simulink model "HILClimbers_Integrated_V7"  (R2021a)
settings: Solver=FixedStepAuto  StartTime=0.0  StopTime=10.0  RelTol=1e-3
undefined symbols (not defined in the file or in its folder): sigbuilder_block
settings Model: VariantConfigurationObject=test_mode  TunableVars=time_period  TunableVarsStorageClass=ExportedGlobal  OrderedModelArguments=off  Creator=achu  LastModifiedBy=achu
settings DebuggingCC: AlgebraicLoopMsg=none

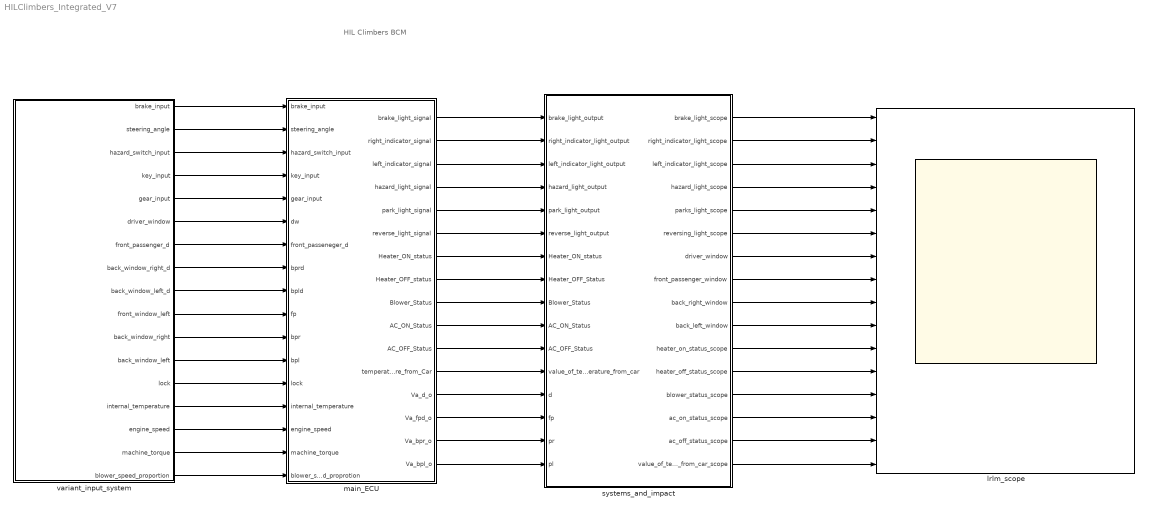
== system HILClimbers_Integrated_V7 ==
  note: HIL Climbers BCM
  lrlm_scope : Scope  NumInputPorts=16
  main_ECU : Subsystem
  systems_and_impact : Subsystem
  variant_input_system : Subsystem  InitFcn=|  Variant=on
      | manual_test=Simulink.Variant("test_mode==0");
      | automated_test=Simulink.Variant("test_mode==1");
  wires:
  systems_and_impact/4(hazard_light_scope) -> lrlm_scope/4
  systems_and_impact/12(heater_off_status_scope) -> lrlm_scope/12
  main_ECU/13(Va_d_o) -> systems_and_impact/13(d)
  systems_and_impact/10(back_left_window) -> lrlm_scope/10
  variant_input_system/6(driver_window) -> main_ECU/6(dw)
  variant_input_system/11(back_window_right) -> main_ECU/11(bpr)
  variant_input_system/9(back_window_left_d) -> main_ECU/9(bpld)
  variant_input_system/1(brake_input) -> main_ECU/1(brake_input)
  variant_input_system/10(front_window_left) -> main_ECU/10(fp)
  variant_input_system/16(machine_torque) -> main_ECU/16(machine_torque)
  variant_input_system/3(hazard_switch_input) -> main_ECU/3(hazard_switch_input)
  main_ECU/8(Heater_OFF_status) -> systems_and_impact/8(Heater_OFF_Status)
  variant_input_system/8(back_window_right_d) -> main_ECU/8(bprd)
  systems_and_impact/13(blower_status_scope) -> lrlm_scope/13
  systems_and_impact/6(reversing_light_scope) -> lrlm_scope/6
  main_ECU/3(left_indicator_signal) -> systems_and_impact/3(left_indicator_light_output)
  main_ECU/2(right_indicator_signal) -> systems_and_impact/2(right_indicator_light_output)
  variant_input_system/17(blower_speed_proportion) -> main_ECU/17(blower_speed_proprotion)
  main_ECU/10(AC_ON_Status) -> systems_and_impact/10(AC_ON_Status)
  variant_input_system/15(engine_speed) -> main_ECU/15(engine_speed)
  main_ECU/12(temperature_from_Car) -> systems_and_impact/12(value_of_temperature_from_car)
  systems_and_impact/11(heater_on_status_scope) -> lrlm_scope/11
  variant_input_system/7(front_passenger_d) -> main_ECU/7(front_passeneger_d)
  variant_input_system/13(lock) -> main_ECU/13(lock)
  systems_and_impact/16(value_of_temperature_from_car_scope) -> lrlm_scope/16
  main_ECU/9(Blower_Status) -> systems_and_impact/9(Blower_Status)
  systems_and_impact/15(ac_off_status_scope) -> lrlm_scope/15
  systems_and_impact/3(left_indicator_light_scope) -> lrlm_scope/3
  main_ECU/4(hazard_light_signal) -> systems_and_impact/4(hazard_light_output)
  main_ECU/16(Va_bpl_o) -> systems_and_impact/16(pl)
  main_ECU/11(AC_OFF_Status) -> systems_and_impact/11(AC_OFF_Status)
  main_ECU/6(reverse_light_signal) -> systems_and_impact/6(reverse_light_output)
  main_ECU/15(Va_bpr_o) -> systems_and_impact/15(pr)
  systems_and_impact/9(back_right_window) -> lrlm_scope/9
  main_ECU/7(Heater_ON_status) -> systems_and_impact/7(Heater_ON_status)
  systems_and_impact/2(right_indicator_light_scope) -> lrlm_scope/2
  variant_input_system/12(back_window_left) -> main_ECU/12(bpl)
  variant_input_system/4(key_input) -> main_ECU/4(key_input)
  systems_and_impact/8(front_passenger_window) -> lrlm_scope/8
  systems_and_impact/1(brake_light_scope) -> lrlm_scope/1
  systems_and_impact/7(driver_window) -> lrlm_scope/7
  main_ECU/1(brake_light_signal) -> systems_and_impact/1(brake_light_output)
  systems_and_impact/5(parks_light_scope) -> lrlm_scope/5
  variant_input_system/2(steering_angle) -> main_ECU/2(steering_angle)
  systems_and_impact/14(ac_on_status_scope) -> lrlm_scope/14
  main_ECU/14(Va_fpd_o) -> systems_and_impact/14(fp)
  variant_input_system/5(gear_input) -> main_ECU/5(gear_input)
  variant_input_system/14(internal_temperature) -> main_ECU/14(internal_temperature)
  main_ECU/5(park_light_signal) -> systems_and_impact/5(park_light_output)

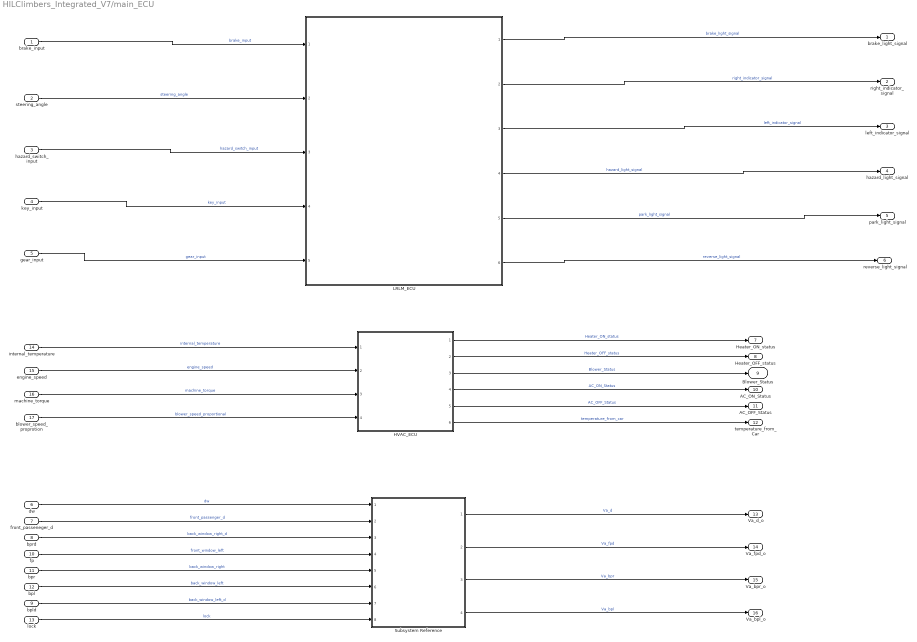
== system HILClimbers_Integrated_V7/main_ECU ==
  brake_input : Inport
  steering_angle : Inport  Port=2
  hazard_switch_input : Inport  Port=3
  key_input : Inport  Port=4
  gear_input : Inport  Port=5
  dw : Inport  Port=6
  front_passeneger_d : Inport  Port=7
  bprd : Inport  Port=8
  bpld : Inport  Port=9
  fp : Inport  Port=10
  bpr : Inport  Port=11
  bpl : Inport  Port=12
  lock : Inport  Port=13
  internal_temperature : Inport  Port=14
  engine_speed : Inport  Port=15
  machine_torque : Inport  Port=16
  blower_speed_proprotion : Inport  Port=17
  HVAC_ECU : Subsystem  ReferencedSubsystem=V6_ECU
  LRLM_ECU : Subsystem  ReferencedSubsystem=LRLM_ECU
  Subsystem Reference : Subsystem  ReferencedSubsystem=power_windows_ECU_V6
  brake_light_signal : Outport
  right_indicator_signal : Outport  Port=2
  left_indicator_signal : Outport  Port=3
  hazard_light_signal : Outport  Port=4
  park_light_signal : Outport  Port=5
  reverse_light_signal : Outport  Port=6
  Heater_ON_status : Outport  Port=7
  Heater_OFF_status : Outport  Port=8
  Blower_Status : Outport  Port=9
  AC_ON_Status : Outport  Port=10
  AC_OFF_Status : Outport  Port=11
  temperature_from_Car : Outport  Port=12
  Va_d_o : Outport  Port=13
  Va_fpd_o : Outport  Port=14
  Va_bpr_o : Outport  Port=15
  Va_bpl_o : Outport  Port=16
  wires:
  HVAC_ECU/1 -> Heater_ON_status/1  "Heater_ON_status"
  hazard_switch_input/1 -> LRLM_ECU/3  "hazard_switch_input"
  LRLM_ECU/1 -> brake_light_signal/1  "brake_light_signal"
  HVAC_ECU/5 -> AC_OFF_Status/1  "AC_OFF_Status"
  steering_angle/1 -> LRLM_ECU/2  "steering_angle"
  LRLM_ECU/2 -> right_indicator_signal/1  "right_indicator_signal"
  LRLM_ECU/5 -> park_light_signal/1  "park_light_signal"
  brake_input/1 -> LRLM_ECU/1  "brake_input"
  engine_speed/1 -> HVAC_ECU/2  "engine_speed"
  LRLM_ECU/3 -> left_indicator_signal/1  "left_indicator_signal"
  LRLM_ECU/4 -> hazard_light_signal/1  "hazard_light_signal"
  internal_temperature/1 -> HVAC_ECU/1  "internal_temperature"
  LRLM_ECU/6 -> reverse_light_signal/1  "reverse_light_signal"
  gear_input/1 -> LRLM_ECU/5  "gear_input"
  HVAC_ECU/2 -> Heater_OFF_status/1  "Heater_OFF_status"
  key_input/1 -> LRLM_ECU/4  "key_input"
  blower_speed_proprotion/1 -> HVAC_ECU/4  "blower_speed_proportional"
  HVAC_ECU/6 -> temperature_from_Car/1  "temperature_from_car"
  HVAC_ECU/4 -> AC_ON_Status/1  "AC_ON_Status"
  machine_torque/1 -> HVAC_ECU/3  "machine_torque"
  HVAC_ECU/3 -> Blower_Status/1  "Blower_Status"
  Subsystem Reference/1 -> Va_d_o/1  "Va_d"
  bpl/1 -> Subsystem Reference/6  "back_window_left"
  Subsystem Reference/3 -> Va_bpr_o/1  "Va_bpr"
  bpld/1 -> Subsystem Reference/7  "back_window_left_d"
  bprd/1 -> Subsystem Reference/3  "back_window_right_d"
  fp/1 -> Subsystem Reference/4  "front_window_left"
  Subsystem Reference/2 -> Va_fpd_o/1  "Va_fpd"
  bpr/1 -> Subsystem Reference/5  "back_window_right"
  dw/1 -> Subsystem Reference/1  "dw"
  Subsystem Reference/4 -> Va_bpl_o/1  "Va_bpl"
  lock/1 -> Subsystem Reference/8  "lock"
  front_passeneger_d/1 -> Subsystem Reference/2  "front_passenger_d"

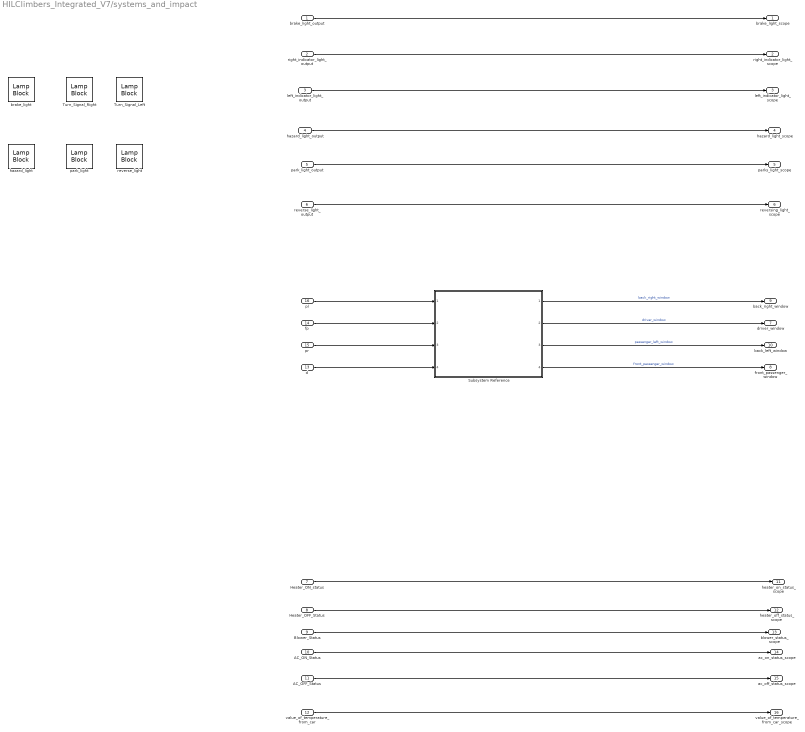
== system HILClimbers_Integrated_V7/systems_and_impact ==
  brake_light_output : Inport
  right_indicator_light_output : Inport  Port=2
  left_indicator_light_output : Inport  Port=3
  hazard_light_output : Inport  Port=4
  park_light_output : Inport  Port=5
  reverse_light_output : Inport  Port=6
  Heater_ON_status : Inport  Port=7
  Heater_OFF_Status : Inport  Port=8
  Blower_Status : Inport  Port=9
  AC_ON_Status : Inport  Port=10
  AC_OFF_Status : Inport  Port=11
  value_of_temperature_from_car : Inport  Port=12
  d : Inport  Port=13
  fp : Inport  Port=14
  pr : Inport  Port=15
  pl : Inport  Port=16
  Subsystem Reference : Subsystem  ReferencedSubsystem=power_window_system_impact_V6
  Turn_Signal_Left : LampBlock  LabelPosition=Hide  Icon=TurnSignalLeft
  Turn_Signal_Right : LampBlock  LabelPosition=Hide  Icon=TurnSignalRight
  brake_light : LampBlock  LabelPosition=Hide  Icon=LightingSwitch
  hazard_light : LampBlock  LabelPosition=Hide  Icon=Hazards
  park_light : LampBlock  LabelPosition=Hide  Icon=ParkingAssistance
  reverse_light : LampBlock  LabelPosition=Hide  Icon=RearFogLight
  brake_light_scope : Outport
  right_indicator_light_scope : Outport  Port=2
  left_indicator_light_scope : Outport  Port=3
  hazard_light_scope : Outport  Port=4
  parks_light_scope : Outport  Port=5
  reversing_light_scope : Outport  Port=6
  driver_window : Outport  Port=7
  front_passenger_window : Outport  Port=8
  back_right_window : Outport  Port=9
  back_left_window : Outport  Port=10
  heater_on_status_scope : Outport  Port=11
  heater_off_status_scope : Outport  Port=12
  blower_status_scope : Outport  Port=13
  ac_on_status_scope : Outport  Port=14
  ac_off_status_scope : Outport  Port=15
  value_of_temperature_from_car_scope : Outport  Port=16
  wires:
  hazard_light_output/1 -> hazard_light_scope/1
  reverse_light_output/1 -> reversing_light_scope/1
  park_light_output/1 -> parks_light_scope/1
  left_indicator_light_output/1 -> left_indicator_light_scope/1
  right_indicator_light_output/1 -> right_indicator_light_scope/1
  brake_light_output/1 -> brake_light_scope/1
  Subsystem Reference/4 -> front_passenger_window/1  "front_passenger_window"
  Subsystem Reference/3 -> back_left_window/1  "passenger_left_window"
  Subsystem Reference/1 -> back_right_window/1  "back_right_window"
  Subsystem Reference/2 -> driver_window/1  "driver_window"
  Blower_Status/1 -> blower_status_scope/1
  AC_OFF_Status/1 -> ac_off_status_scope/1
  AC_ON_Status/1 -> ac_on_status_scope/1
  Heater_OFF_Status/1 -> heater_off_status_scope/1
  Heater_ON_status/1 -> heater_on_status_scope/1
  value_of_temperature_from_car/1 -> value_of_temperature_from_car_scope/1
  pl/1 -> Subsystem Reference/1
  fp/1 -> Subsystem Reference/2
  d/1 -> Subsystem Reference/4
  pr/1 -> Subsystem Reference/3

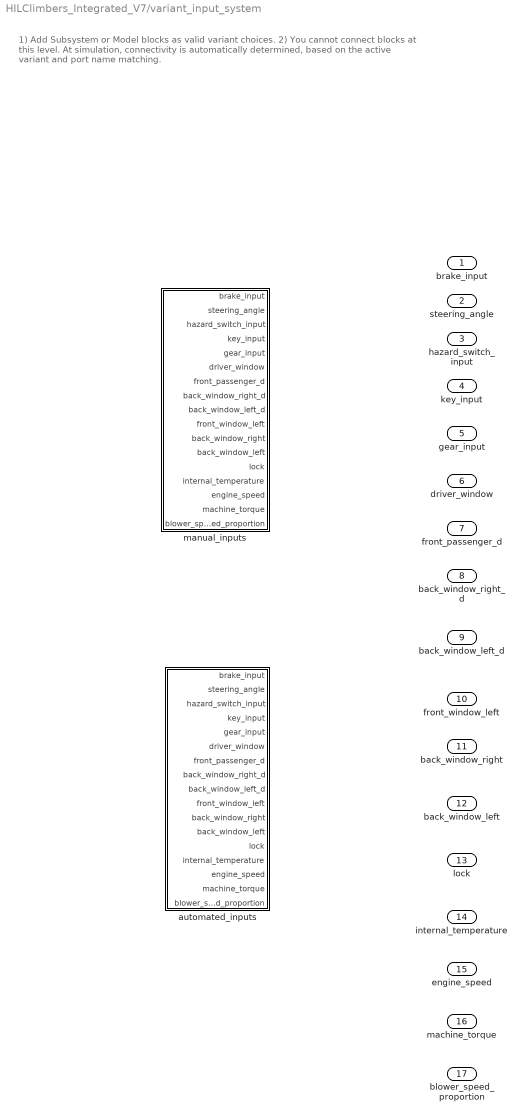
== system HILClimbers_Integrated_V7/variant_input_system ==
  note: 1) Add Subsystem or Model blocks as valid variant choices.
      | 2) You cannot connect blocks at this level. At simulation, connectivity is automatically
      | determined, based on the active variant and port name matching.
  automated_inputs : Subsystem  VariantControl=automated_test
  manual_inputs : Subsystem  VariantControl=manual_test
  brake_input : Outport
  steering_angle : Outport  Port=2
  hazard_switch_input : Outport  Port=3
  key_input : Outport  Port=4
  gear_input : Outport  Port=5
  driver_window : Outport  Port=6
  front_passenger_d : Outport  Port=7
  back_window_right_d : Outport  Port=8
  back_window_left_d : Outport  Port=9
  front_window_left : Outport  Port=10
  back_window_right : Outport  Port=11
  back_window_left : Outport  Port=12
  lock : Outport  Port=13
  internal_temperature : Outport  Port=14
  engine_speed : Outport  Port=15
  machine_torque : Outport  Port=16
  blower_speed_proportion : Outport  Port=17

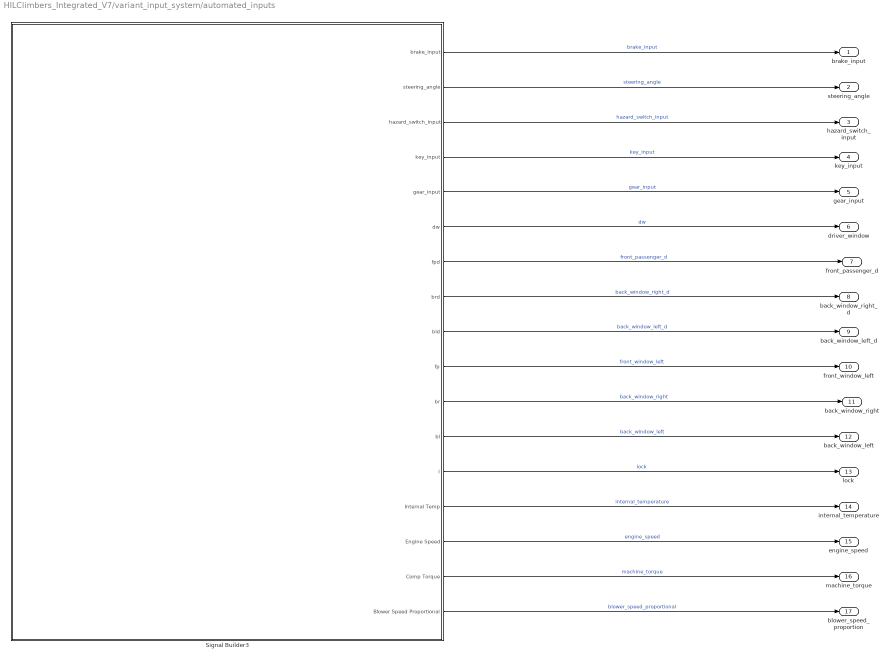
== system HILClimbers_Integrated_V7/variant_input_system/automated_inputs ==
  Signal Builder3 : Subsystem  Tag=STV Subsys  LoadFcn=sigbuilder_block('load');  StartFcn=sigbuilder_block('start');  StopFcn=sigbuilder_block('stop');  ClipboardFcn=sigbuilder_block('clipboard');  mask(Sigbuilder block){tuvar=[0:10]}
      mask help: Simulink:masks:SigbuilderBlock_MD
      mask init:
      | if ~strcmp(get_param(bdroot(gcbh),'SimulationStatus'),'stopped') tuvar = sigbuilder_block('maskInit'); end
      settings: CopyFcn=sigbuilder_block('copy');  DeleteFcn=sigbuilder_block('delete');  ModelCloseFcn=sigbuilder_block('modelClose');  PreSaveFcn=sigbuilder_block('preSave');  PauseFcn=sigbuilder_block('pause');  ContinueFcn=sigbuilder_block('continue');  NameChangeFcn=sigbuilder_block('namechange');  OpenFcn=sigbuilder_block('open',[437.6 199.2 550.4 400 ]);  CloseFcn=sigbuilder_block('close');
      mask Display: plot(0, 0, 100, 100,[2, 2, 32, 32, 2], [68, 8, 8, 68, 68],[32, 2], [38, 38], [32, 19, 2],[53, 60, 44], [32, 17, 17, 2],[16, 16, 31, 31]);txt = getActiveGroup(gcbh);text(2, 100, txt,'verticalAlignment', 'top');
  brake_input : Outport
  steering_angle : Outport  Port=2
  hazard_switch_input : Outport  Port=3
  key_input : Outport  Port=4
  gear_input : Outport  Port=5
  driver_window : Outport  Port=6
  front_passenger_d : Outport  Port=7
  back_window_right_d : Outport  Port=8
  back_window_left_d : Outport  Port=9
  front_window_left : Outport  Port=10
  back_window_right : Outport  Port=11
  back_window_left : Outport  Port=12
  lock : Outport  Port=13
  internal_temperature : Outport  Port=14
  engine_speed : Outport  Port=15
  machine_torque : Outport  Port=16
  blower_speed_proportion : Outport  Port=17
  wires:
  Signal Builder3/11(br) -> back_window_right/1  "back_window_right"
  Signal Builder3/2(steering_angle) -> steering_angle/1  "steering_angle"
  Signal Builder3/13(l) -> lock/1  "lock"
  Signal Builder3/16(Comp Torque) -> machine_torque/1  "machine_torque"
  Signal Builder3/10(fp) -> front_window_left/1  "front_window_left"
  Signal Builder3/5(gear_input) -> gear_input/1  "gear_input"
  Signal Builder3/12(bl) -> back_window_left/1  "back_window_left"
  Signal Builder3/17(Blower Speed Proportional) -> blower_speed_proportion/1  "blower_speed_proportional"
  Signal Builder3/8(brd) -> back_window_right_d/1  "back_window_right_d"
  Signal Builder3/14(Internal Temp) -> internal_temperature/1  "internal_temperature"
  Signal Builder3/3(hazard_switch_input) -> hazard_switch_input/1  "hazard_switch_input"
  Signal Builder3/6(dw) -> driver_window/1  "dw"
  Signal Builder3/1(brake_input) -> brake_input/1  "brake_input"
  Signal Builder3/7(fpd) -> front_passenger_d/1  "front_passenger_d"
  Signal Builder3/9(bld) -> back_window_left_d/1  "back_window_left_d"
  Signal Builder3/15(Engine Speed) -> engine_speed/1  "engine_speed"
  Signal Builder3/4(key_input) -> key_input/1  "key_input"

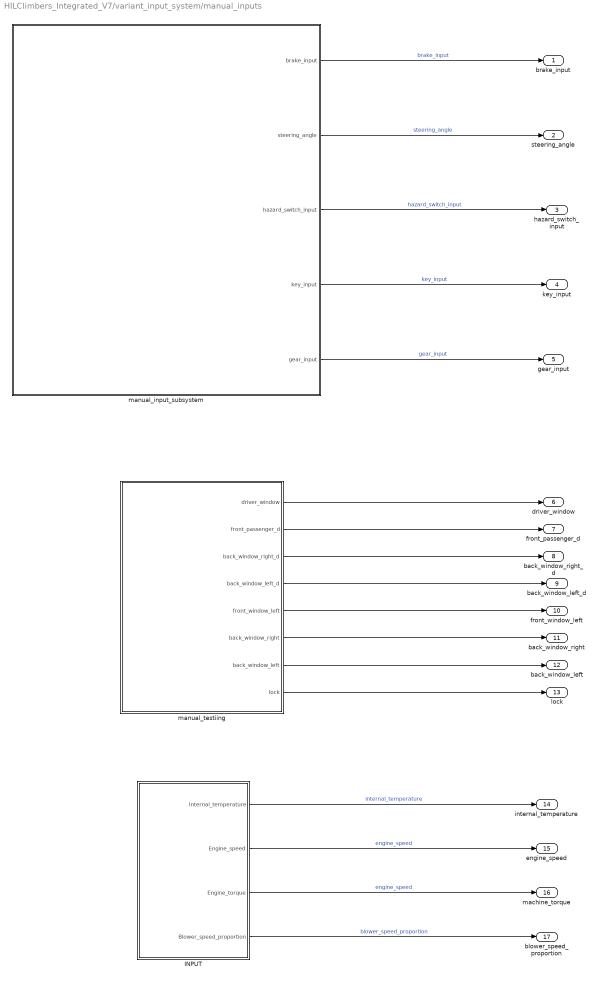
== system HILClimbers_Integrated_V7/variant_input_system/manual_inputs ==
  INPUT : Subsystem
  manual_input_subsystem : Subsystem  VariantControl=manual_test
  manual_testiing : Subsystem  VariantControl=Choice
  brake_input : Outport
  steering_angle : Outport  Port=2
  hazard_switch_input : Outport  Port=3
  key_input : Outport  Port=4
  gear_input : Outport  Port=5
  driver_window : Outport  Port=6
  front_passenger_d : Outport  Port=7
  back_window_right_d : Outport  Port=8
  back_window_left_d : Outport  Port=9
  front_window_left : Outport  Port=10
  back_window_right : Outport  Port=11
  back_window_left : Outport  Port=12
  lock : Outport  Port=13
  internal_temperature : Outport  Port=14
  engine_speed : Outport  Port=15
  machine_torque : Outport  Port=16
  blower_speed_proportion : Outport  Port=17
  wires:
  manual_input_subsystem/3(hazard_switch_input) -> hazard_switch_input/1  "hazard_switch_input"
  manual_input_subsystem/2(steering_angle) -> steering_angle/1  "steering_angle"
  manual_input_subsystem/4(key_input) -> key_input/1  "key_input"
  manual_testiing/1(driver_window) -> driver_window/1
  manual_input_subsystem/1(brake_input) -> brake_input/1  "brake_input"
  manual_testiing/6(back_window_right) -> back_window_right/1
  manual_testiing/5(front_window_left) -> front_window_left/1
  manual_input_subsystem/5(gear_input) -> gear_input/1  "gear_input"
  manual_testiing/3(back_window_right_d) -> back_window_right_d/1
  INPUT/1(Internal_temperature) -> internal_temperature/1  "internal_temperature"
  manual_testiing/8(lock) -> lock/1
  INPUT/3(Engine_torque) -> machine_torque/1  "engine_speed"
  manual_testiing/4(back_window_left_d) -> back_window_left_d/1
  INPUT/2(Engine_speed) -> engine_speed/1  "engine_speed"
  manual_testiing/2(front_passenger_d) -> front_passenger_d/1
  INPUT/4(Blower_speed_proportion) -> blower_speed_proportion/1  "blower_speed_proportion"
  manual_testiing/7(back_window_left) -> back_window_left/1

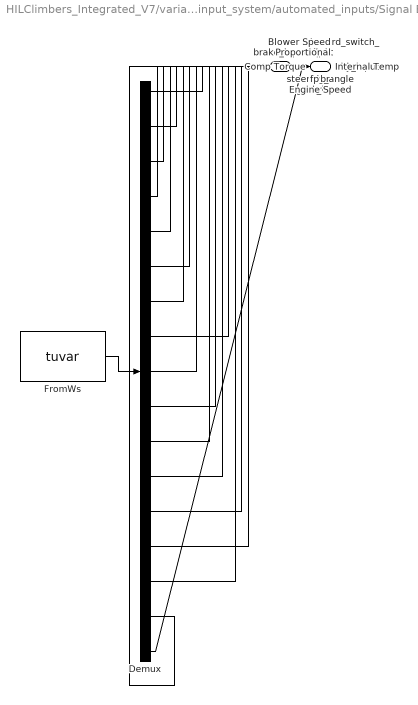
== system HILClimbers_Integrated_V7/variant_input_system/automated_inputs/Signal Builder3 ==
  Demux : Demux  Tag=STV Demux  Outputs=17
      settings: DisplayOption=none
  FromWs : FromWorkspace  Tag=STV FromWs  VariableName=tuvar
      SigBuilderData=|
      | common.afterFinalStr = 'Extrapolate'
      | common.sampleTime = 0
      | dataSet.timeRange = [0 20]
      | dataSet.name = 'Sheet1'
      | sbobj.Name = 'Signal Builder'
      | sbobj.Groups.Name = 'Sheet1'
      | sbobj.Groups.Signals(1).Name = 'brake_input'
      | sbobj.Groups.Signals(1).XData = [0 1 2 3 4 5 6 7 8 9 10 11 12 13 14 15 16 17 18 19 20]
      | sbobj.Groups.Signals(1).YData = [0 0 0 0 0 0 0 0 0 0 0 1 1 1 1 1 1 1 1 1 1]
      | sbobj.Groups.Signals(2).Name = 'steering_angle'
      | sbobj.Groups.Signals(2).XData = [0 1 2 3 4 5 6 7 8 9 10 11 12 13 14 15 16 17 18 19 20]
      | sbobj.Groups.Signals(2).YData = [-45 -45 -45 -45 -45 -45 -45 -45 0 0 0 0 0 0 0 0 45 45 45 45 45]
      | sbobj.Groups.Signals(3).Name = 'hazard_switch_input'
      | sbobj.Groups.Signals(3).XData = [0 1 2 3 4 5 6 7 8 9 10 11 12 13 14 15 16 17 18 19 20]
      | sbobj.Groups.Signals(3).YData = [0 0 0 0 0 0 0 0 0 0 0 0 0 0 0 0 1 1 1 1 1]
      | sbobj.Groups.Signals(4).Name = 'key_input'
      | sbobj.Groups.Signals(4).XData = [0 1 2 3 4 5 6 7 8 9 10 11 12 13 14 15 16 17 18 19 20]
      | sbobj.Groups.Signals(4).YData = [0 0 0 0 0 0 0 0 1 1 1 1 1 1 1 1 0 0 0 0 0]
      | sbobj.Groups.Signals(5).Name = 'gear_input'
      | sbobj.Groups.Signals(5).XData = [0 1 2 3 4 5 6 7 8 9 10 11 12 13 14 15 16 17 18 19 20]
      | sbobj.Groups.Signals(5).YData = [0 0 1 1 2 2 3 3 0 0 1 1 2 2 3 3 0 0 1 1 1]
      | sbobj.Groups.Signals(6).Name = 'dw'
      | sbobj.Groups.Signals(6).XData = [0 1 2 3 4 5 6 7 8 9 10 11 12 13 14 15 16 17 18 19 20]
      | sbobj.Groups.Signals(6).YData = [0 1 1 1 0 0 0 0 -1 -1 -1 -1 -1 1 1 1 1 0 0 0 0]
      | sbobj.Groups.Signals(7).Name = 'fpd'
      | sbobj.Groups.Signals(7).XData = [0 1 2 3 4 5 6 7 8 9 10 11 12 13 14 15 16 17 18 19 20]
      | sbobj.Groups.Signals(7).YData = [0 1 1 -1 -1 -1 1 1 1 1 1 0 0 0 0 0 0 0 0 0 0]
      | sbobj.Groups.Signals(8).Name = 'brd'
      | sbobj.Groups.Signals(8).XData = [0 1 2 3 4 5 6 7 8 9 10 11 12 13 14 15 16 17 18 19 20]
      | sbobj.Groups.Signals(8).YData = [0 1 1 1 1 -1 -1 -1 -1 -1 -1 0 0 0 0 0 0 0 0 0 0]
      | sbobj.Groups.Signals(9).Name = 'bld'
      | sbobj.Groups.Signals(9).XData = [0 1 2 3 4 5 6 7 8 9 10 11 12 13 14 15 16 17 18 19 20]
      | sbobj.Groups.Signals(9).YData = [0 1 1 1 1 -1 -1 -1 -1 -1 1 1 1 0 0 0 0 0 0 0 0]
      | sbobj.Groups.Signals(10).Name = 'fp'
      | sbobj.Groups.Signals(10).XData = [0 1 2 3 4 5 6 7 8 9 10 11 12 13 14 15 16 17 18 19 20]
      | sbobj.Groups.Signals(10).YData = [0 -1 -1 1 1 1 -1 -1 -1 -1 -1 -1 -1 -1 1 1 1 1 1 1 1]
      | sbobj.Groups.Signals(11).Name = 'br'
      | sbobj.Groups.Signals(11).XData = [0 1 2 3 4 5 6 7 8 9 10 11 12 13 14 15 16 17 18 19 20]
      | sbobj.Groups.Signals(11).YData = [0 -1 -1 -1 -1 1 1 -1 -1 1 1 1 1 -1 -1 -1 -1 1 1 1 1]
      | sbobj.Groups.Signals(12).Name = 'bl'
      | sbobj.Groups.Signals(12).XData = [0 1 2 3 4 5 6 7 8 9 10 11 12 13 14 15 16 17 18 19 20]
      | sbobj.Groups.Signals(12).YData = [0 1 1 0 0 1 1 0 0 1 1 -1 -1 -1 -1 -1 -1 1 1 1 1]
      | sbobj.Groups.Signals(13).Name = 'l'
      | sbobj.Groups.Signals(13).XData = [0 1 2 3 4 5 6 7 8 9 10 11 12 13 14 15 16 17 18 19 20]
      | sbobj.Groups.Signals(13).YData = [0 0 0 0 0 0 1 1 1 1 1 1 1 1 0 0 0 0 0 0 0]
      | sbobj.Groups.Signals(14).Name = 'Internal Temp'
      | sbobj.Groups.Signals(14).XData = [0 1 2 3 4 5 6 7 8 9 10 11 12 13 14 15 16 17 18 19 20]
      | sbobj.Groups.Signals(14).YData = [5 10 15 20 25 30 30 5 10 15 20 25 30 30 5 10 15 20 25 30 30]
      | sbobj.Groups.Signals(15).Name = 'Engine Speed'
      | sbobj.Groups.Signals(15).XData = [0 1 2 3 4 5 6 7 8 9 10 11 12 13 14 15 16 17 18 19 20]
      | sbobj.Groups.Signals(15).YData = [0 20 40 60 80 100 120 0 20 40 60 80 100 120 0 20 40 60 80 100 120]
      | sbobj.Groups.Signals(16).Name = 'Comp Torque'
      | sbobj.Groups.Signals(16).XData = [0 1 2 3 4 5 6 7 8 9 10 11 12 13 14 15 16 17 18 19 20]
      | sbobj.Groups.Signals(16).YData = [5 10 15 20 25 30 30 5 10 15 20 25 30 30 5 10 15 20 25 30 30]
      | sbobj.Groups.Signals(17).Name = 'Blower Speed Proportional'
      | sbobj.Groups.Signals(17).XData = [0 1 2 3 4 5 6 7 8 9 10 11 12 13 14 15 16 17 18 19 20]
      | sbobj.Groups.Signals(17).YData = [2 2 4 6 8 10 12 2 2 4 6 8 10 12 2 2 4 6 8 10 12]
      | sbobj.Groups.TimeRange = [0 20]
  brake_input : Outport  Tag=STV Outport
  steering_angle : Outport  Tag=STV Outport  Port=2
  hazard_switch_input : Outport  Tag=STV Outport  Port=3
  key_input : Outport  Tag=STV Outport  Port=4
  gear_input : Outport  Tag=STV Outport  Port=5
  dw : Outport  Tag=STV Outport  Port=6
  fpd : Outport  Tag=STV Outport  Port=7
  brd : Outport  Tag=STV Outport  Port=8
  bld : Outport  Tag=STV Outport  Port=9
  fp : Outport  Tag=STV Outport  Port=10
  br : Outport  Tag=STV Outport  Port=11
  bl : Outport  Tag=STV Outport  Port=12
  l : Outport  Tag=STV Outport  Port=13
  Internal Temp : Outport  Tag=STV Outport  Port=14
  Engine Speed : Outport  Tag=STV Outport  Port=15
  Comp Torque : Outport  Tag=STV Outport  Port=16
  Blower Speed Proportional : Outport  Tag=STV Outport  Port=17
  wires:
  Demux/1 -> brake_input/1
  FromWs/1 -> Demux/1
  Demux/2 -> steering_angle/1
  Demux/3 -> hazard_switch_input/1
  Demux/4 -> key_input/1
  Demux/5 -> gear_input/1
  Demux/6 -> dw/1
  Demux/7 -> fpd/1
  Demux/8 -> brd/1
  Demux/9 -> bld/1
  Demux/10 -> fp/1
  Demux/11 -> br/1
  Demux/12 -> bl/1
  Demux/13 -> l/1
  Demux/14 -> Internal Temp/1
  Demux/15 -> Engine Speed/1
  Demux/16 -> Comp Torque/1
  Demux/17 -> Blower Speed Proportional/1

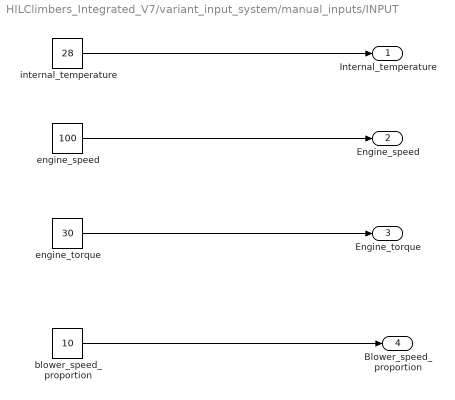
== system HILClimbers_Integrated_V7/variant_input_system/manual_inputs/INPUT ==
  blower_speed_proportion : Constant  Value=10
  engine_speed : Constant  Value=100
  engine_torque : Constant  Value=30
  internal_temperature : Constant  Value=28
  Internal_temperature : Outport
  Engine_speed : Outport  Port=2
  Engine_torque : Outport  Port=3
  Blower_speed_proportion : Outport  Port=4
  wires:
  internal_temperature/1 -> Internal_temperature/1
  engine_torque/1 -> Engine_torque/1
  blower_speed_proportion/1 -> Blower_speed_proportion/1
  engine_speed/1 -> Engine_speed/1

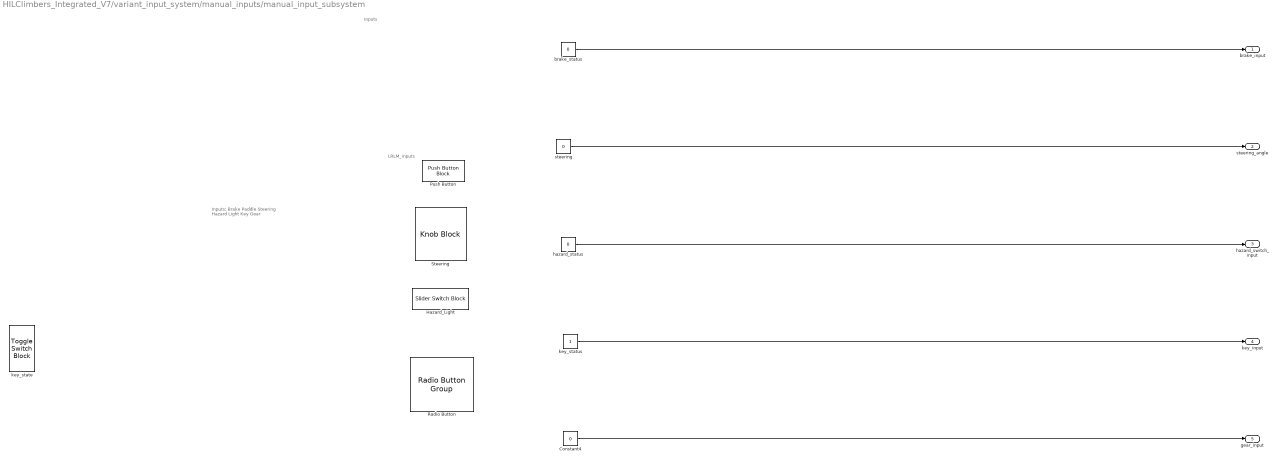
== system HILClimbers_Integrated_V7/variant_input_system/manual_inputs/manual_input_subsystem ==
  note: Inputs
  note: LRLM_inputs
  note: Inputs:
      | Brake Paddle
      | Steering
      | Hazard Light
      | Key
      | Gear
  Constant4 : Constant  Value=0
  Hazard_Light : SliderSwitchBlock  LabelPosition=Hide
      settings: Values={{'Off', 'On'}, [0 1]}
  Push Button : PushButtonBlock  ButtonText=Brake
  Radio Button : RadioButtonGroup  LabelPosition=Hide  SelectedLabel=Neutral  ButtonGroupName=Gear
      settings: Values={{'Neutral', 'Drive', 'Park', 'Reverse'}, [0 1 2 3]}
  Steering : KnobBlock  LabelPosition=Hide  ScaleMin=-90  ScaleMax=90  TickInterval=45
  brake_status : Constant  Value=0
  hazard_status : Constant  Value=0
  key_state : ToggleSwitchBlock  LabelPosition=Bottom
      settings: Values={{'Off', 'On'}, [0 1]}
  key_status : Constant
  steering : Constant  Value=0
  brake_input : Outport
  steering_angle : Outport  Port=2
  hazard_switch_input : Outport  Port=3
  key_input : Outport  Port=4
  gear_input : Outport  Port=5
  wires:
  brake_status/1 -> brake_input/1
  Constant4/1 -> gear_input/1
  steering/1 -> steering_angle/1
  key_status/1 -> key_input/1
  hazard_status/1 -> hazard_switch_input/1

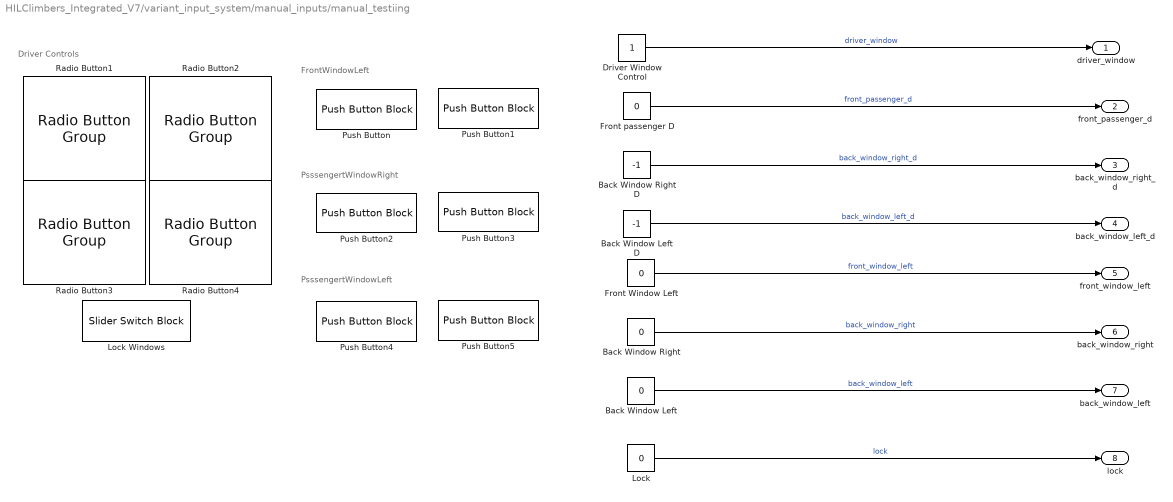
== system HILClimbers_Integrated_V7/variant_input_system/manual_inputs/manual_testiing ==
  note: PsssengertWindowLeft
  note: PsssengertWindowRight
  note: Driver Controls
  note: FrontWindowLeft
  Back Window Left : Constant  Value=0
  Back Window Left D : Constant  Value=-1
  Back Window Right : Constant  Value=0
  Back Window Right D : Constant  Value=-1
  Driver Window Control : Constant
  Front Window Left : Constant  Value=0
  Front passenger D : Constant  Value=0
  Lock : Constant  Value=0
  Lock Windows : SliderSwitchBlock
      settings: Values={{'Unlock', 'Lock'}, [0 1]}
  Push Button : PushButtonBlock  ButtonText=Push up window
  Push Button1 : PushButtonBlock  ButtonText=Pull down window  OnValue=-1
  Push Button2 : PushButtonBlock  ButtonText=Push up window
  Push Button3 : PushButtonBlock  ButtonText=Pull down window  OnValue=-1
  Push Button4 : PushButtonBlock  ButtonText=Push up window
  Push Button5 : PushButtonBlock  ButtonText=Pull down window  OnValue=-1
  Radio Button1 : RadioButtonGroup  LabelPosition=Hide  SelectedLabel=Open  ButtonGroupName=Driver Window Controls
      settings: Values={{'Open', 'Stop', 'Close'}, [1 0 -1]}
  Radio Button2 : RadioButtonGroup  LabelPosition=Hide  SelectedLabel=Stop  ButtonGroupName=Front Passenger
      settings: Values={{'Open', 'Stop', 'Close'}, [1 0 -1]}
  Radio Button3 : RadioButtonGroup  LabelPosition=Hide  SelectedLabel=Close  ButtonGroupName=Back Window Right
      settings: Values={{'Open', 'Stop', 'Close'}, [1 0 -1]}
  Radio Button4 : RadioButtonGroup  LabelPosition=Hide  SelectedLabel=Close  ButtonGroupName=Back Window Left
      settings: Values={{'Open', 'Stop', 'Close'}, [1 0 -1]}
  driver_window : Outport
  front_passenger_d : Outport  Port=2
  back_window_right_d : Outport  Port=3
  back_window_left_d : Outport  Port=4
  front_window_left : Outport  Port=5
  back_window_right : Outport  Port=6
  back_window_left : Outport  Port=7
  lock : Outport  Port=8
  wires:
  Front passenger D/1 -> front_passenger_d/1  "front_passenger_d"
  Lock/1 -> lock/1  "lock"
  Front Window Left/1 -> front_window_left/1  "front_window_left"
  Driver Window Control/1 -> driver_window/1  "driver_window"
  Back Window Right D/1 -> back_window_right_d/1  "back_window_right_d"
  Back Window Left/1 -> back_window_left/1  "back_window_left"
  Back Window Right/1 -> back_window_right/1  "back_window_right"
  Back Window Left D/1 -> back_window_left_d/1  "back_window_left_d"
